simulink library "libraryProject2"  (R2017a)
settings: Solver=VariableStepAuto  StartTime=0.0  StopTime=10.0  RelTol=1e-3
libraries: realtime_pacer_lib x1
settings Model: Creator=ibrahim  LastModifiedBy=ibrahim

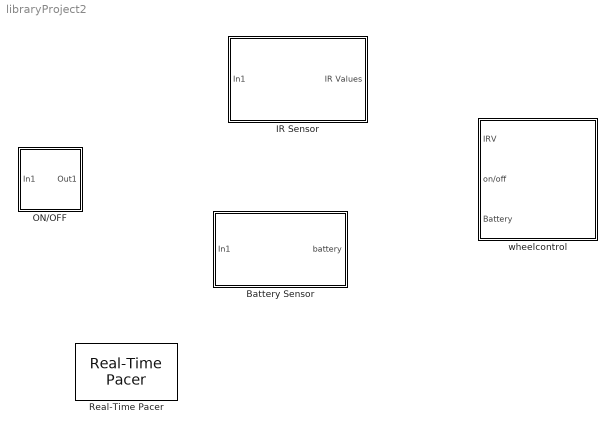
== system libraryProject2 ==
  Battery Sensor : Subsystem
  IR Sensor : Subsystem
  ON/OFF : Subsystem
  Real-Time Pacer : realtime_pacer_lib/Real-Time Pacer  simTimePerRealTime=.5
  wheelcontrol : Subsystem

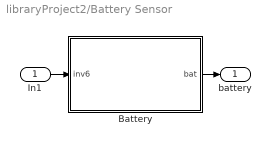
== system libraryProject2/Battery Sensor ==
  In1 : Inport
  Battery : Stateflow chart  TreatAsAtomicUnit=on
  battery : Outport
  wires:
  In1/1 -> Battery/1(inv6)
  Battery/1(bat) -> battery/1

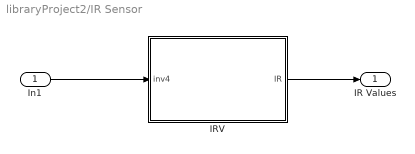
== system libraryProject2/IR Sensor ==
  In1 : Inport
  IRV : Stateflow chart  TreatAsAtomicUnit=on
  IR Values : Outport
  wires:
  In1/1 -> IRV/1(inv4)
  IRV/1(IR) -> IR Values/1

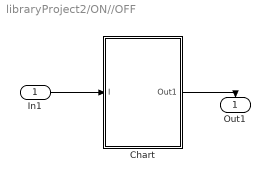
== system libraryProject2/ON//OFF ==
  In1 : Inport
  Chart : Stateflow chart  TreatAsAtomicUnit=on
  Out1 : Outport
  wires:
  Chart/1(Out1) -> Out1/1
  In1/1 -> Chart/1(I)

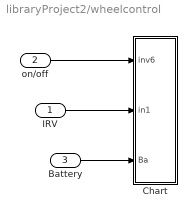
== system libraryProject2/wheelcontrol ==
  IRV : Inport
  on/off : Inport  Port=2
  Battery : Inport  Port=3
  Chart : Stateflow chart  TreatAsAtomicUnit=on
  wires:
  on/off/1 -> Chart/1(inv6)
  Battery/1 -> Chart/3(Ba)
  IRV/1 -> Chart/2(in1)

== stateflow chart libraryProject2/Battery Sensor/Battery ==
  state wait
    en,du:
  state on
    en,du:
    bat=battery;
  state off
    en,du:
    bat=0;
  wait -> on : after(60,sec)
  on -> wait [order 2] : after(.5,sec)
  (default) -> off
  off -> on : [inv6==1]
  on -> off [order 1] : [inv6==0]
  data: y function_output; inv6 input; bat output
  function y=battery:
    | function y=battery
    | persistent so5
    | y=0;
    | coder.extrinsic('evalin');
    | coder.extrinsic('get');
    | so5 = evalin('base','ha');
    | B=0;
    | coder.extrinsic('BatteryChargeReaderRoomba_me');
    | B= BatteryChargeReaderRoomba_me(so5);
    | y=B;

== stateflow chart libraryProject2/ON//OFF/Chart ==
  state init
    en:
    tcpinit;
    Out1=1;
  state TurnRoombaOff
    en:
    OFF;
    Out1=0;
  (default) -> init
  TurnRoombaOff -> init : [I==1]
  init -> TurnRoombaOff : [I==0]
  data: Out1 output; I input
  function tcpinit:
    | function tcpinit
    | coder.extrinsic('RoombaInit_wifi');
    | coder.extrinsic('assignin');
    | persistent tcpobj
    | tcpobj=RoombaInit_wifi('10.0.0.1','full');
    | assignin('base','ha',tcpobj);
  function OFF:
    | function OFF
    | persistent sl
    | 
    | coder.extrinsic('evalin');
    | coder.extrinsic('get');
    | sl = evalin('base','ha');
    | coder.extrinsic('PowerOffRoomba')
    | PowerOffRoomba(sl);

== stateflow chart libraryProject2/IR Sensor/IRV ==
  state on
    en,du:
    IR=IRV;
  state off
    en,du:
    IR=zeros(1,6);
  (default) -> off
  off -> on : [inv4==1]
  on -> off : [inv4==0]
  data: y function_output; IR output; inv4 input
  function y= IRV:
    | function y= IRV
    | persistent so1
    | y=zeros(1,6);
    | coder.extrinsic('evalin');
    | 
    |     so1 = evalin('base','ha');
    | 
    | IR = zeros(1, 6);
    | coder.extrinsic('RangeStateRoomba');
    | IR = RangeStateRoomba(so1);
    | y=IR;

== stateflow chart libraryProject2/wheelcontrol/Chart ==
  state on1
    state off
      en,du:
      AutoControl(0,0);
    state on
      state reverseabit
        entry:
        AutoControl(-.1,-0.1);
      state gostraight
        entry,du:
        AutoControl(0.05,0.05);
      state turnrightinplace
        entry,du:
        AutoControl(-0.2,0.2);
      state turnleftinplace
        entry,du:
        AutoControl(0.2,-0.2);
      state turnleft
        entry,du:
        AutoControl(0.2,-0.2);
      state turnright
        entry,du:
        AutoControl(-0.2,0.2);
      state turnleft1
        entry,du:
        AutoControl(.2,-0.2);
      state turnright1
        entry,du:
        AutoControl(-0.2,.2);
      (default) -> reverseabit
      reverseabit -> gostraight : after(1,sec)
      gostraight -> turnright1 [order 1] : [in1(1)>0]
      turnright1 -> gostraight : [in1(1)<1]
      gostraight -> turnright [order 2] : [in1(2)>0]
      turnright -> gostraight : [in1(2)<1]
      gostraight -> turnrightinplace [order 3] : [in1(3)>0]
      turnrightinplace -> gostraight : [in1(3)<1]
      gostraight -> turnleftinplace [order 4] : [in1(4)>0]
      turnleftinplace -> gostraight : [in1(4)<1]
      gostraight -> turnleft [order 5] : [in1(5)>0]
      turnleft -> gostraight : [in1(5)<1]
      gostraight -> turnleft1 [order 6] : [in1(6)>0]
      turnleft1 -> gostraight : [in1(6)<1]
    (default) -> on1.off
    on1.off -> on : [Ba>=3]
    on -> on1.off : [Ba<=2]
  state off
    en,du:
  (default) -> off
  off -> on1 : [inv6==1]
  on1 -> off : [inv6==0]
  data: u1 function_input; u2 function_input; inv6 input; in1 input; Ba input
  function AutoControl(u1,u2):
    | function AutoControl(u1,u2)
    | persistent so
    | coder.extrinsic('evalin');
    | coder.extrinsic('get');
    | so = evalin('base','ha');
    | coder.extrinsic('SetWheelVelRoomba');
    | SetWheelVelRoomba(so,u1 , u2);
